simulink model "lab3_hugo"  (R2022a)
settings: Solver=VariableStepAuto  StartTime=0.0  StopTime=60000  RelTol=1e-3
undefined symbols (not defined in the file or in its folder): T
settings Model: Creator=hugoa  LastModifiedBy=hugoa

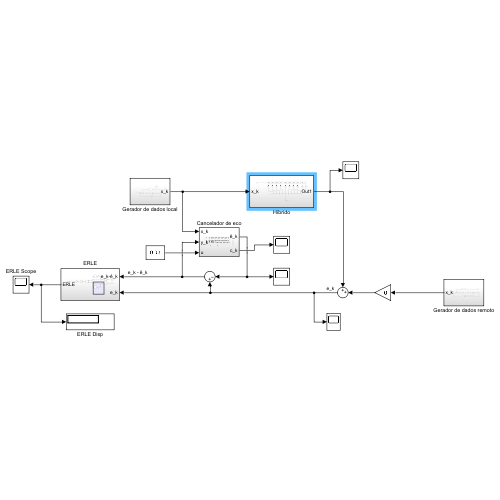
[thumbnail: Simulink's stored preview of the top-level diagram]
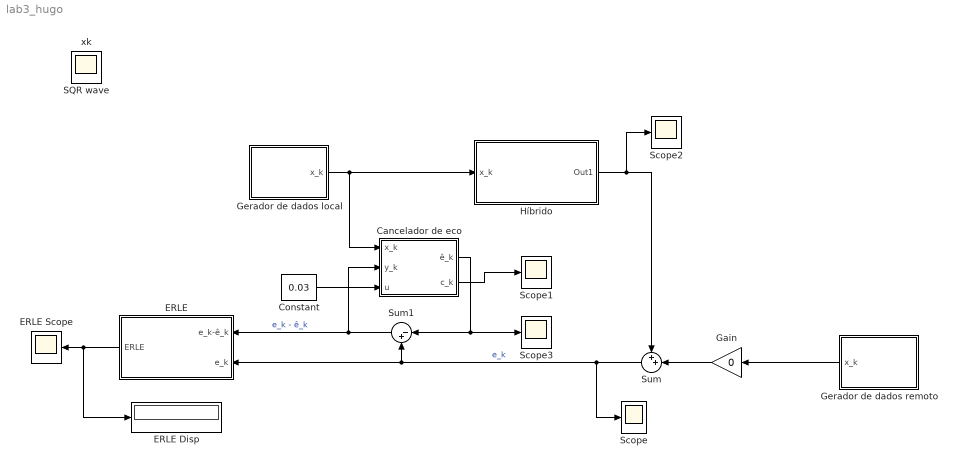
== system lab3_hugo ==
  Cancelador de eco : Subsystem
  Constant : Constant  Value=0.03
  ERLE : Subsystem
  ERLE Disp : Display
  ERLE Scope : Scope
  Gain : Gain  Gain=0
  Gerador de dados local : Subsystem
  Gerador de dados remoto : Subsystem
  Híbrido : Subsystem
  Scope{,1..3} (4 alike) : Scope
  Sum : Sum  Inputs=++|
  Sum1 : Sum  Inputs=|-+
  SQR wave : Scope
  xk : Scope
  wires:
  Gerador de dados local/1(x_k) -> Híbrido/1(x_k), Cancelador de eco/1(x_k)
  Gerador de dados remoto/1(x_k) -> Gain/1
  Gain/1 -> Sum/2
  Híbrido/1(Out1) -> Scope2/1, Sum/1
  Sum/1 -> Scope/1, ERLE/2(e_k), Sum1/2  "e_k"
  Sum1/1 -> ERLE/1(e_k-ê_k), Cancelador de eco/2(y_k)  "e_k - ê_k"
  ERLE/1(ERLE) -> ERLE Disp/1, ERLE Scope/1
  Cancelador de eco/2(c_k) -> Scope1/1
  Constant/1 -> Cancelador de eco/3(u)
  Cancelador de eco/1(ê_k) -> Scope3/1, Sum1/1

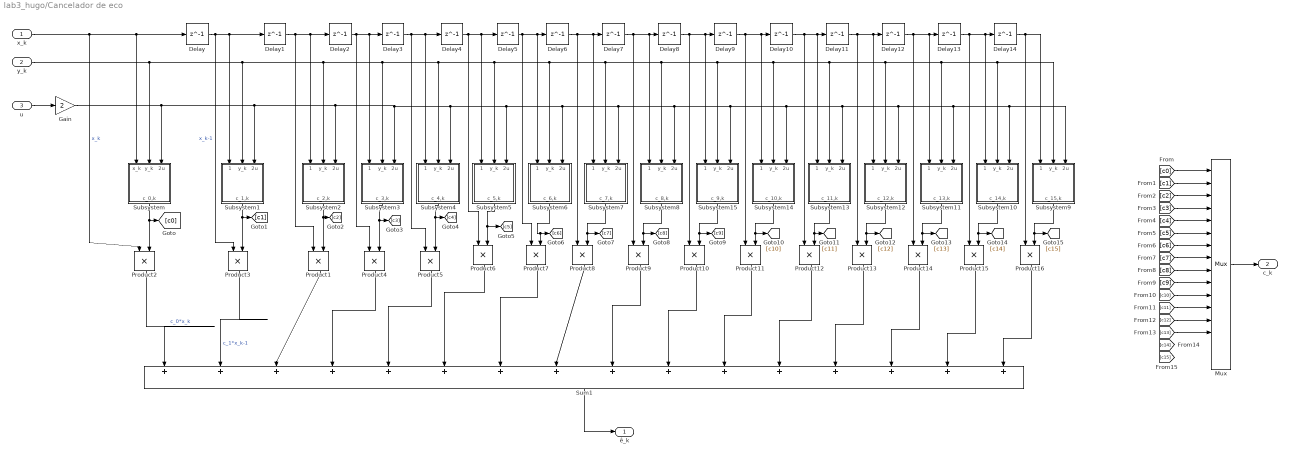
== system lab3_hugo/Cancelador de eco ==
  x_k : Inport
  y_k : Inport  Port=2
  u : Inport  Port=3
  Delay{,1..14} (15 alike) : Delay  DelayLength=1  SampleTime=T
  Gain : Gain  Gain=2
  Mux : Mux  Inputs=16
      settings: DisplayOption=signals
  Product{1..16} (16 alike) : Product
  Subsystem : Subsystem
  Subsystem1 : Subsystem
  Subsystem10 : Subsystem
  Subsystem11 : Subsystem
  Subsystem12 : Subsystem
  Subsystem13 : Subsystem
  Subsystem14 : Subsystem
  Subsystem15 : Subsystem
  Subsystem2 : Subsystem
  Subsystem3 : Subsystem
  Subsystem4 : Subsystem
  Subsystem5 : Subsystem
  Subsystem6 : Subsystem
  Subsystem7 : Subsystem
  Subsystem8 : Subsystem
  Subsystem9 : Subsystem
  Sum1 : Sum  Inputs=|++++++++++++++++
  ê_k : Outport
  c_k : Outport  Port=2
  wires:
  x_k/1 -> Product2/1, Delay/1, Subsystem/1(x_k)  "x_k"
  Delay/1 -> Delay1/1, Subsystem1/1(x_k-1), Product3/1  "x_k-1"
  Product2/1 -> Sum1/1  "c_0*x_k"
  Product3/1 -> Sum1/2  "c_1*x_k-1"
  Sum1/1 -> ê_k/1
  Subsystem1/1(c_1,k) -> Product3/2, [c1]
  Delay1/1 -> Product1/1, Delay2/1, Subsystem2/1(x_k-2)
  Gain/1 -> Subsystem5/3(2u), Subsystem6/3(2u), Subsystem7/3(2u), Subsystem8/3(2u), Subsystem15/3(2u), Subsystem14/3(2u), Subsystem13/3(2u), Subsystem12/3(2u), Subsystem11/3(2u), Subsystem10/3(2u), Subsystem9/3(2u), Subsystem4/3(2u), Subsystem3/3(2u), Subsystem2/3(2u), Subsystem1/3(2u), Subsystem/3(2u)
  Subsystem2/1(c_2,k) -> [c2], Product1/2
  Product1/1 -> Sum1/3
  Subsystem3/1(c_3,k) -> [c3], Product4/2
  Subsystem4/1(c_4,k) -> [c4], Product5/2
  Product4/1 -> Sum1/4
  Product5/1 -> Sum1/5
  Delay2/1 -> Product4/1, Delay3/1, Subsystem3/1(x_k-3)
  Delay3/1 -> Delay4/1, Subsystem4/1(x_k-4), Product5/1
  Product6/1 -> Sum1/6
  Product7/1 -> Sum1/7
  Product8/1 -> Sum1/8
  Product9/1 -> Sum1/9
  Product10/1 -> Sum1/10
  Product11/1 -> Sum1/11
  Product12/1 -> Sum1/12
  Product13/1 -> Sum1/13
  Product14/1 -> Sum1/14
  Product15/1 -> Sum1/15
  Product16/1 -> Sum1/16
  Subsystem5/1(c_5,k) -> Product6/2, [c5]
  Delay4/1 -> Product6/1, Delay5/1, Subsystem5/1(x_k-5)
  y_k/1 -> Subsystem13/2(y_k), Subsystem9/2(y_k), Subsystem10/2(y_k), Subsystem11/2(y_k), Subsystem12/2(y_k), Subsystem14/2(y_k), Subsystem15/2(y_k), Subsystem8/2(y_k), Subsystem7/2(y_k), Subsystem6/2(y_k), Subsystem5/2(y_k), Subsystem4/2(y_k), Subsystem3/2(y_k), Subsystem2/2(y_k), Subsystem1/2(y_k), Subsystem/2(y_k)
  Delay5/1 -> Delay6/1, Subsystem6/1(x_k-6), Product7/1
  Delay6/1 -> Delay7/1, Subsystem7/1(x_k-7), Product8/1
  Delay7/1 -> Delay8/1, Subsystem8/1(x_k-8), Product9/1
  Subsystem6/1(c_6,k) -> [c6], Product7/2
  Subsystem7/1(c_7,k) -> [c7], Product8/2
  Subsystem8/1(c_8,k) -> [c8], Product9/2
  Delay8/1 -> Delay9/1, Subsystem15/1(x_k-9), Product10/1
  Subsystem15/1(c_9,k) -> [c9], Product10/2
  Delay9/1 -> Subsystem14/1(x_k-10), Delay10/1, Product11/1
  Subsystem14/1(c_10,k) -> [c10], Product11/2
  Delay10/1 -> Delay11/1, Subsystem13/1(x_k-11), Product12/1
  Delay11/1 -> Subsystem12/1(x_k-12), Delay12/1, Product13/1
  Delay12/1 -> Product14/1, Subsystem11/1(x_k-13), Delay13/1
  Delay13/1 -> Subsystem10/1(x_k-14), Delay14/1, Product15/1
  Subsystem12/1(c_12,k) -> [c12], Product13/2
  Subsystem11/1(c_13,k) -> [c13], Product14/2
  Subsystem10/1(c_14,k) -> [c14], Product15/2
  Subsystem9/1(c_15,k) -> [c15], Product16/2
  Delay14/1 -> Subsystem9/1(x_k-15), Product16/1
  Subsystem13/1(c_11,k) -> [c11], Product12/2
  Subsystem/1(c_0,k) -> [c0], Product2/2
  [c0] -> Mux/1
  [c1] -> Mux/2
  [c9] -> Mux/10
  [c8] -> Mux/9
  [c7] -> Mux/8
  [c6] -> Mux/7
  [c5] -> Mux/6
  [c4] -> Mux/5
  [c3] -> Mux/4
  [c2] -> Mux/3
  [c10] -> Mux/11
  [c11] -> Mux/12
  [c12] -> Mux/13
  [c13] -> Mux/14
  Mux/1 -> c_k/1
  u/1 -> Gain/1

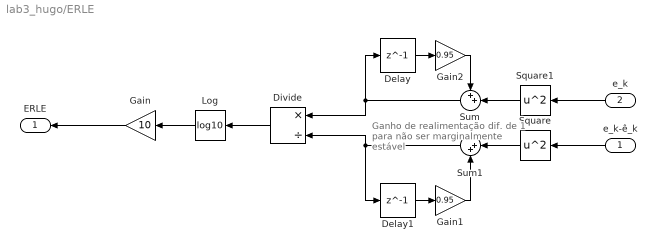
== system lab3_hugo/ERLE ==
  note: Ganho de realimentação
      | dif. de 1 para não ser
      | marginalmente estável
  e_k-ê_k : Inport
  e_k : Inport  Port=2
  Delay : Delay  DelayLength=1  SampleTime=T
  Delay1 : Delay  DelayLength=1  SampleTime=T
  Divide : Product  Inputs=*/
  Gain : Gain  Gain=10
  Gain1 : Gain  Gain=0.95
  Gain2 : Gain  Gain=0.95
  Log : Math  Operator=log10
  Square : Math  Operator=square
  Square1 : Math  Operator=square
  Sum : Sum  Inputs=++|
  Sum1 : Sum  Inputs=|++
  ERLE : Outport
  wires:
  Square1/1 -> Sum/2
  Sum1/1 -> Delay1/1, Divide/2
  Delay1/1 -> Gain1/1
  Sum/1 -> Delay/1, Divide/1
  e_k/1 -> Square1/1
  Square/1 -> Sum1/1
  e_k-ê_k/1 -> Square/1
  Log/1 -> Gain/1
  Gain1/1 -> Sum1/2
  Gain2/1 -> Sum/1
  Divide/1 -> Log/1
  Delay/1 -> Gain2/1
  Gain/1 -> ERLE/1

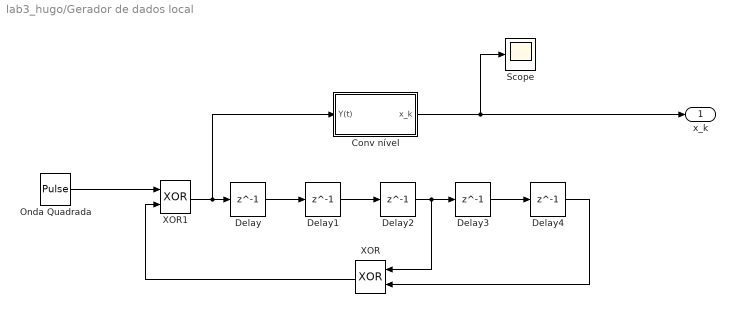
== system lab3_hugo/Gerador de dados local ==
  Conv nível : Subsystem
  Delay{,1..4} (5 alike) : Delay  DelayLength=1  SampleTime=T
  Onda Quadrada : DiscretePulseGenerator  PulseType=Time based  Period=T  PulseWidth=50
  Scope : Scope
  XOR : Logic  Operator=XOR  AllPortsSameDT=off  OutDataTypeStr=boolean
  XOR1 : Logic  Operator=XOR  AllPortsSameDT=off  OutDataTypeStr=boolean
  x_k : Outport
  wires:
  Delay1/1 -> Delay2/1
  Onda Quadrada/1 -> XOR1/1
  Delay3/1 -> Delay4/1
  Delay2/1 -> XOR/1, Delay3/1
  Conv nível/1(x_k) -> Scope/1, x_k/1
  XOR1/1 -> Conv nível/1(Y(t)), Delay/1
  Delay4/1 -> XOR/2
  Delay/1 -> Delay1/1
  XOR/1 -> XOR1/2

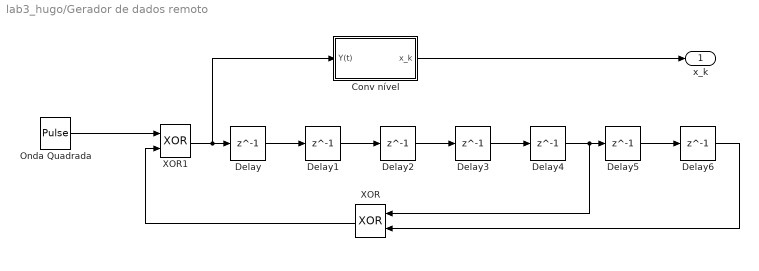
== system lab3_hugo/Gerador de dados remoto ==
  Conv nível : Subsystem
  Delay{,1..6} (7 alike) : Delay  DelayLength=1  SampleTime=T
  Onda Quadrada : DiscretePulseGenerator  PulseType=Time based  Period=2*T  PulseWidth=50
  XOR : Logic  Operator=XOR  AllPortsSameDT=off  OutDataTypeStr=boolean
  XOR1 : Logic  Operator=XOR  AllPortsSameDT=off  OutDataTypeStr=boolean
  x_k : Outport
  wires:
  XOR/1 -> XOR1/2
  Delay/1 -> Delay1/1
  XOR1/1 -> Delay/1, Conv nível/1(Y(t))
  Conv nível/1(x_k) -> x_k/1
  Delay2/1 -> Delay3/1
  Delay3/1 -> Delay4/1
  Onda Quadrada/1 -> XOR1/1
  Delay1/1 -> Delay2/1
  Delay4/1 -> Delay5/1, XOR/1
  Delay5/1 -> Delay6/1
  Delay6/1 -> XOR/2

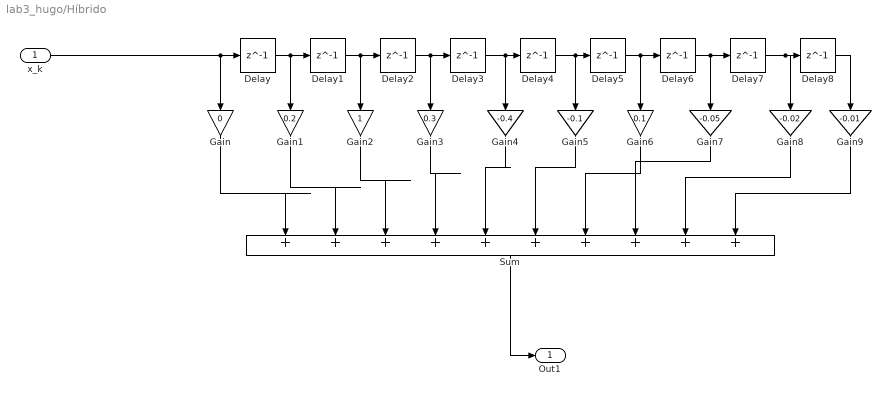
== system lab3_hugo/Híbrido ==
  x_k : Inport
  Delay{,1..8} (9 alike) : Delay  DelayLength=1  SampleTime=T
  Gain : Gain  Gain=0
  Gain1 : Gain  Gain=0.2
  Gain2 : Gain
  Gain3 : Gain  Gain=0.3
  Gain4 : Gain  Gain=-0.4
  Gain5 : Gain  Gain=-0.1
  Gain6 : Gain  Gain=0.1
  Gain7 : Gain  Gain=-0.05
  Gain8 : Gain  Gain=-0.02
  Gain9 : Gain  Gain=-0.01
  Sum : Sum  Inputs=|++++++++++
  Out1 : Outport
  wires:
  Delay5/1 -> Gain6/1, Delay6/1
  x_k/1 -> Delay/1, Gain/1
  Delay4/1 -> Gain5/1, Delay5/1
  Gain6/1 -> Sum/7
  Delay1/1 -> Delay2/1, Gain2/1
  Gain5/1 -> Sum/6
  Gain9/1 -> Sum/10
  Delay/1 -> Delay1/1, Gain1/1
  Delay2/1 -> Gain3/1, Delay3/1
  Gain/1 -> Sum/1
  Gain7/1 -> Sum/8
  Gain3/1 -> Sum/4
  Gain4/1 -> Sum/5
  Delay8/1 -> Gain9/1
  Delay3/1 -> Delay4/1, Gain4/1
  Delay7/1 -> Gain8/1, Delay8/1
  Gain2/1 -> Sum/3
  Delay6/1 -> Delay7/1, Gain7/1
  Gain1/1 -> Sum/2
  Gain8/1 -> Sum/9
  Sum/1 -> Out1/1

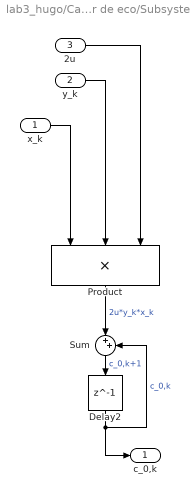
== system lab3_hugo/Cancelador de eco/Subsystem ==
  x_k : Inport
  y_k : Inport  Port=2
  2u : Inport  Port=3
  Delay2 : Delay  DelayLength=1  SampleTime=T
  Product : Product  Inputs=3
  Sum : Sum  Inputs=|++
  c_0,k : Outport
  wires:
  y_k/1 -> Product/2
  Product/1 -> Sum/1  "2u*y_k*x_k"
  Sum/1 -> Delay2/1  "c_0,k+1"
  Delay2/1 -> c_0,k/1, Sum/2  "c_0,k"
  x_k/1 -> Product/1
  2u/1 -> Product/3

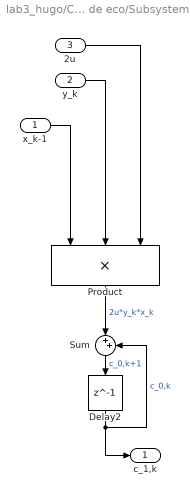
== system lab3_hugo/Cancelador de eco/Subsystem1 ==
  x_k-1 : Inport
  y_k : Inport  Port=2
  2u : Inport  Port=3
  Delay2 : Delay  DelayLength=1  SampleTime=T
  Product : Product  Inputs=3
  Sum : Sum  Inputs=|++
  c_1,k : Outport
  wires:
  y_k/1 -> Product/2
  Product/1 -> Sum/1  "2u*y_k*x_k"
  Sum/1 -> Delay2/1  "c_0,k+1"
  Delay2/1 -> c_1,k/1, Sum/2  "c_0,k"
  x_k-1/1 -> Product/1
  2u/1 -> Product/3

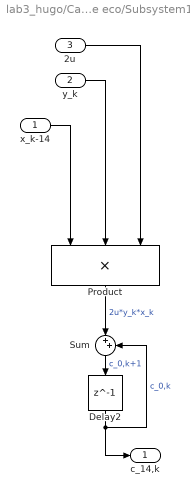
== system lab3_hugo/Cancelador de eco/Subsystem10 ==
  x_k-14 : Inport
  y_k : Inport  Port=2
  2u : Inport  Port=3
  Delay2 : Delay  DelayLength=1
  Product : Product  Inputs=3
  Sum : Sum  Inputs=|++
  c_14,k : Outport
  wires:
  2u/1 -> Product/3
  x_k-14/1 -> Product/1
  Delay2/1 -> Sum/2, c_14,k/1  "c_0,k"
  Sum/1 -> Delay2/1  "c_0,k+1"
  Product/1 -> Sum/1  "2u*y_k*x_k"
  y_k/1 -> Product/2

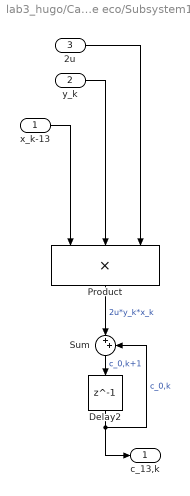
== system lab3_hugo/Cancelador de eco/Subsystem11 ==
  x_k-13 : Inport
  y_k : Inport  Port=2
  2u : Inport  Port=3
  Delay2 : Delay  DelayLength=1
  Product : Product  Inputs=3
  Sum : Sum  Inputs=|++
  c_13,k : Outport
  wires:
  2u/1 -> Product/3
  x_k-13/1 -> Product/1
  Delay2/1 -> Sum/2, c_13,k/1  "c_0,k"
  Sum/1 -> Delay2/1  "c_0,k+1"
  Product/1 -> Sum/1  "2u*y_k*x_k"
  y_k/1 -> Product/2

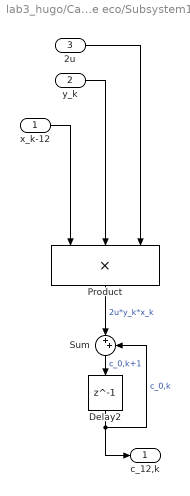
== system lab3_hugo/Cancelador de eco/Subsystem12 ==
  x_k-12 : Inport
  y_k : Inport  Port=2
  2u : Inport  Port=3
  Delay2 : Delay  DelayLength=1
  Product : Product  Inputs=3
  Sum : Sum  Inputs=|++
  c_12,k : Outport
  wires:
  2u/1 -> Product/3
  x_k-12/1 -> Product/1
  Delay2/1 -> Sum/2, c_12,k/1  "c_0,k"
  Sum/1 -> Delay2/1  "c_0,k+1"
  Product/1 -> Sum/1  "2u*y_k*x_k"
  y_k/1 -> Product/2

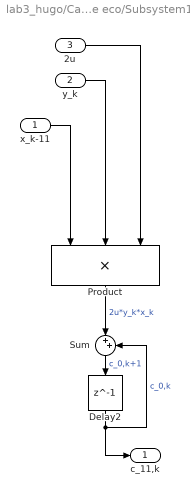
== system lab3_hugo/Cancelador de eco/Subsystem13 ==
  x_k-11 : Inport
  y_k : Inport  Port=2
  2u : Inport  Port=3
  Delay2 : Delay  DelayLength=1
  Product : Product  Inputs=3
  Sum : Sum  Inputs=|++
  c_11,k : Outport
  wires:
  2u/1 -> Product/3
  x_k-11/1 -> Product/1
  Delay2/1 -> Sum/2, c_11,k/1  "c_0,k"
  Sum/1 -> Delay2/1  "c_0,k+1"
  Product/1 -> Sum/1  "2u*y_k*x_k"
  y_k/1 -> Product/2

== system lab3_hugo/Cancelador de eco/Subsystem14 ==
  x_k-10 : Inport
  y_k : Inport  Port=2
  2u : Inport  Port=3
  Delay2 : Delay  DelayLength=1
  Product : Product  Inputs=3
  Sum : Sum  Inputs=|++
  c_10,k : Outport
  wires:
  2u/1 -> Product/3
  x_k-10/1 -> Product/1
  Delay2/1 -> Sum/2, c_10,k/1  "c_0,k"
  Sum/1 -> Delay2/1  "c_0,k+1"
  Product/1 -> Sum/1  "2u*y_k*x_k"
  y_k/1 -> Product/2

== system lab3_hugo/Cancelador de eco/Subsystem15 ==
  x_k-9 : Inport
  y_k : Inport  Port=2
  2u : Inport  Port=3
  Delay2 : Delay  DelayLength=1
  Product : Product  Inputs=3
  Sum : Sum  Inputs=|++
  c_9,k : Outport
  wires:
  2u/1 -> Product/3
  x_k-9/1 -> Product/1
  Delay2/1 -> Sum/2, c_9,k/1  "c_0,k"
  Sum/1 -> Delay2/1  "c_0,k+1"
  Product/1 -> Sum/1  "2u*y_k*x_k"
  y_k/1 -> Product/2

== system lab3_hugo/Cancelador de eco/Subsystem2 ==
  x_k-2 : Inport
  y_k : Inport  Port=2
  2u : Inport  Port=3
  Delay2 : Delay  DelayLength=1
  Product : Product  Inputs=3
  Sum : Sum  Inputs=|++
  c_2,k : Outport
  wires:
  2u/1 -> Product/3
  x_k-2/1 -> Product/1
  Delay2/1 -> Sum/2, c_2,k/1  "c_0,k"
  Sum/1 -> Delay2/1  "c_0,k+1"
  Product/1 -> Sum/1  "2u*y_k*x_k"
  y_k/1 -> Product/2

== system lab3_hugo/Cancelador de eco/Subsystem3 ==
  x_k-3 : Inport
  y_k : Inport  Port=2
  2u : Inport  Port=3
  Delay2 : Delay  DelayLength=1
  Product : Product  Inputs=3
  Sum : Sum  Inputs=|++
  c_3,k : Outport
  wires:
  2u/1 -> Product/3
  x_k-3/1 -> Product/1
  Delay2/1 -> Sum/2, c_3,k/1  "c_0,k"
  Sum/1 -> Delay2/1  "c_0,k+1"
  Product/1 -> Sum/1  "2u*y_k*x_k"
  y_k/1 -> Product/2

== system lab3_hugo/Cancelador de eco/Subsystem4 ==
  x_k-4 : Inport
  y_k : Inport  Port=2
  2u : Inport  Port=3
  Delay2 : Delay  DelayLength=1
  Product : Product  Inputs=3
  Sum : Sum  Inputs=|++
  c_4,k : Outport
  wires:
  2u/1 -> Product/3
  x_k-4/1 -> Product/1
  Delay2/1 -> Sum/2, c_4,k/1  "c_0,k"
  Sum/1 -> Delay2/1  "c_0,k+1"
  Product/1 -> Sum/1  "2u*y_k*x_k"
  y_k/1 -> Product/2

== system lab3_hugo/Cancelador de eco/Subsystem5 ==
  x_k-5 : Inport
  y_k : Inport  Port=2
  2u : Inport  Port=3
  Delay2 : Delay  DelayLength=1
  Product : Product  Inputs=3
  Sum : Sum  Inputs=|++
  c_5,k : Outport
  wires:
  2u/1 -> Product/3
  x_k-5/1 -> Product/1
  Delay2/1 -> Sum/2, c_5,k/1  "c_0,k"
  Sum/1 -> Delay2/1  "c_0,k+1"
  Product/1 -> Sum/1  "2u*y_k*x_k"
  y_k/1 -> Product/2

== system lab3_hugo/Cancelador de eco/Subsystem6 ==
  x_k-6 : Inport
  y_k : Inport  Port=2
  2u : Inport  Port=3
  Delay2 : Delay  DelayLength=1
  Product : Product  Inputs=3
  Sum : Sum  Inputs=|++
  c_6,k : Outport
  wires:
  2u/1 -> Product/3
  x_k-6/1 -> Product/1
  Delay2/1 -> Sum/2, c_6,k/1  "c_0,k"
  Sum/1 -> Delay2/1  "c_0,k+1"
  Product/1 -> Sum/1  "2u*y_k*x_k"
  y_k/1 -> Product/2

== system lab3_hugo/Cancelador de eco/Subsystem7 ==
  x_k-7 : Inport
  y_k : Inport  Port=2
  2u : Inport  Port=3
  Delay2 : Delay  DelayLength=1
  Product : Product  Inputs=3
  Sum : Sum  Inputs=|++
  c_7,k : Outport
  wires:
  2u/1 -> Product/3
  x_k-7/1 -> Product/1
  Delay2/1 -> Sum/2, c_7,k/1  "c_0,k"
  Sum/1 -> Delay2/1  "c_0,k+1"
  Product/1 -> Sum/1  "2u*y_k*x_k"
  y_k/1 -> Product/2

== system lab3_hugo/Cancelador de eco/Subsystem8 ==
  x_k-8 : Inport
  y_k : Inport  Port=2
  2u : Inport  Port=3
  Delay2 : Delay  DelayLength=1
  Product : Product  Inputs=3
  Sum : Sum  Inputs=|++
  c_8,k : Outport
  wires:
  2u/1 -> Product/3
  x_k-8/1 -> Product/1
  Delay2/1 -> Sum/2, c_8,k/1  "c_0,k"
  Sum/1 -> Delay2/1  "c_0,k+1"
  Product/1 -> Sum/1  "2u*y_k*x_k"
  y_k/1 -> Product/2

== system lab3_hugo/Cancelador de eco/Subsystem9 ==
  x_k-15 : Inport
  y_k : Inport  Port=2
  2u : Inport  Port=3
  Delay2 : Delay  DelayLength=1
  Product : Product  Inputs=3
  Sum : Sum  Inputs=|++
  c_15,k : Outport
  wires:
  2u/1 -> Product/3
  x_k-15/1 -> Product/1
  Delay2/1 -> Sum/2, c_15,k/1  "c_0,k"
  Sum/1 -> Delay2/1  "c_0,k+1"
  Product/1 -> Sum/1  "2u*y_k*x_k"
  y_k/1 -> Product/2

== system lab3_hugo/Gerador de dados local/Conv nível ==
  Y(t) : Inport
  Constant : Constant  Value=0.5
  Gain : Gain  Gain=2  OutDataTypeStr=double
  Sum : Sum  Inputs=|+-
  x_k : Outport
  wires:
  Y(t)/1 -> Sum/1
  Sum/1 -> Gain/1
  Constant/1 -> Sum/2
  Gain/1 -> x_k/1

== system lab3_hugo/Gerador de dados remoto/Conv nível ==
  Y(t) : Inport
  Constant : Constant  Value=0.5
  Gain : Gain  Gain=2  OutDataTypeStr=double
  Sum : Sum  Inputs=|+-
  x_k : Outport
  wires:
  Gain/1 -> x_k/1
  Constant/1 -> Sum/2
  Sum/1 -> Gain/1
  Y(t)/1 -> Sum/1
